simulink model "car_control_customAction"  (R2023a)
settings: Solver=VariableStepAuto  StartTime=0.0  StopTime=20  RelTol=1e-3
settings Model: Creator=15113  LastModifiedBy=15113

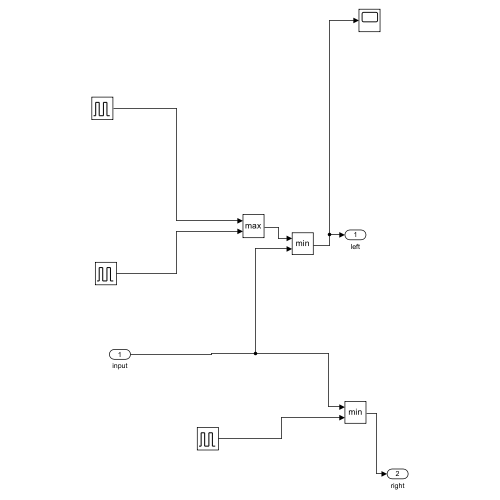
[thumbnail: Simulink's stored preview of the top-level diagram]
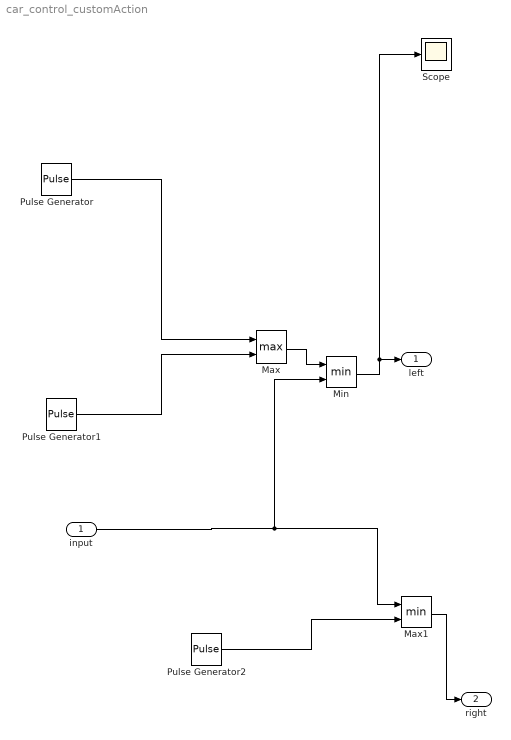
== system car_control_customAction ==
  input : Inport
  Max : MinMax  Function=max  Inputs=2
  Max1 : MinMax  Inputs=2
  Min : MinMax  Inputs=2
  Pulse Generator : DiscretePulseGenerator  PulseType=Time based  Period=50  PulseWidth=80
  Pulse Generator1 : DiscretePulseGenerator  PulseType=Time based  Period=50  PulseWidth=10  PhaseDelay=42.5
  Pulse Generator2 : DiscretePulseGenerator  PulseType=Time based  Period=50  PulseWidth=80
  Scope : Scope
  left : Outport
  right : Outport  Port=2
  wires:
  Pulse Generator1/1 -> Max/2
  Pulse Generator/1 -> Max/1
  input/1 -> Min/2, Max1/1
  Pulse Generator2/1 -> Max1/2
  Max1/1 -> right/1
  Min/1 -> Scope/1, left/1
  Max/1 -> Min/1
